simulink model "Engine"  (R2020a)
settings: Solver=VariableStepAuto  StartTime=0.0  StopTime=10.0  RelTol=1e-3
undefined symbols (not defined in the file or in its folder): breakpoints1, table_data
settings Model: DataDictionary=Properties.sldd  Creator=yafta  LastModifiedBy=Matthew
settings ModelReferenceCC: ModelReferenceMinAlgLoopOccurrences=on

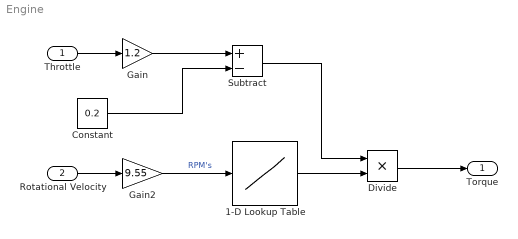
== system Engine ==
  Throttle : Inport
  Rotational Velocity : Inport  Port=2
  1-D Lookup Table : Lookup_n-D  NumberOfTableDimensions=1  BreakpointsForDimension1=breakpoints1  BreakpointsForDimension1DataTypeStr=double  Table=table_data  TableDataTypeStr=double  IntermediateResultsDataTypeStr=double  InternalRulePriority=Speed  OutDataTypeStr=double  RndMeth=Simplest  FractionDataTypeStr=double  InputSameDT=on
  Constant : Constant  Value=0.2
  Divide : Product  Inputs=**
  Gain : Gain  Gain=1.2
  Gain2 : Gain  Gain=9.55
  Subtract : Sum  Inputs=+-
  Torque : Outport
  wires:
  Divide/1 -> Torque/1
  Rotational Velocity/1 -> Gain2/1
  1-D Lookup Table/1 -> Divide/2
  Gain2/1 -> 1-D Lookup Table/1  "RPM's"
  Throttle/1 -> Gain/1
  Constant/1 -> Subtract/2
  Subtract/1 -> Divide/1
  Gain/1 -> Subtract/1
